simulink library "Trajectory"  (R2016a)
settings: Solver=ode45  StartTime=0.0  StopTime=10.0  RelTol=1e-3
settings Model: Creator=Felipe  LastModifiedBy=md13acp
settings DataIOCC: LimitDataPoints=on  SaveFormat=Array
settings DebuggingCC: UnderspecifiedInitializationDetection=Classic  MergeDetectMultiDrivingBlocksExec=none  SolverPrmCheckMsg=warning  StateNameClashWarn=warning
settings HardwareCC: ProdBitPerPointer=32  ProdLargestAtomicFloat=None  ProdIntDivRoundTo=Undefined  ProdEndianess=Unspecified  ProdWordSize=32  ProdHWDeviceType=32-bit Generic
settings ModelReferenceCC: PropagateSignalLabelsOutOfModel=off
settings ConfigComp: CovModelRefEnable=Off

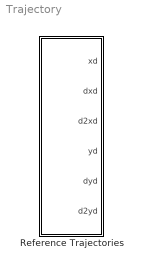
== system Trajectory ==
  Reference Trajectories : Subsystem  mask(Reference Trajectories){trajectory_type=2, wf=0.10, raio_ref_1=1, delta_raio=-0.1, t_delta_raio=60, xd=[2, 3]}
      mask prompts: trajectory_type "Trajectory type: 1=Circle, 2=Eight, 3=Line, 4=Fixed Point"; wf "Angular speed for circle and eight [rad/s]"; raio_ref_1 "Radius for circle and eight (each side) [m]"; delta_raio "Radius variation (circle only)"; t_delta_raio "Time between radius variation (circle only) [s]"; xd "Goal position (for fixed point only) (1x2)"
      mask help: Generates reference values of position, velocity and acceleration.
      mask Help:
      | Generates reference values of position, velocity and acceleration.
      | This block is intended to be used with mobile robot trajectory tracking kinematic controller.
      | 
      | Available references:
      | - Circular trajectory with 2 different radius;
      | - Eight-shape trajectory;
      | - Linear trajectory;
      | - Fixed point.
      | 
      | 
      | <b> Parameters:</b>
      | 
      | Trajectory type: 1=Circle, 2=Eight, 3=Line, 4=Fixed Point
      | Angular speed for circle and eight (1x1) [rad/s]
      | Radius for circle and eight (each side) (1x1)[m]
      | Radius variation (circle only) delta_raio (1x1) [m]
      | Time between radius variation (circle only) (1x1) [s]
      | 
      | <b> Outputs: </b>
      | 
      | xd: desired robot position [m] in x axis;
      | dxd: desired robot speed [m/s] in x axis;
      | d2xd: desired robot acceleration [m/s^2] in x axis;
      | yd: desired robot position [m] in y axis;
      | dyd: desired robot speed [m/s] in y axis;
      | d2yd: desired robot acceleration [m/s^2] in y axis;

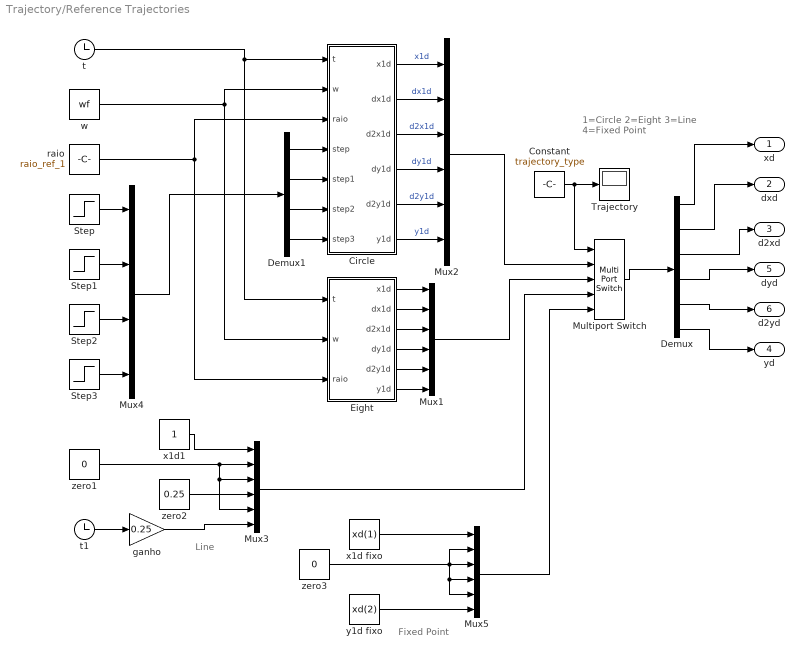
== system Trajectory/Reference Trajectories ==
  note: Fixed Point
  note: Line
  note: 1=Circle
      | 2=Eight
      | 3=Line
      | 4=Fixed Point
  Circle : Subsystem
  Constant : Constant  Value=trajectory_type
  Demux : Demux  Outputs=6
  Demux1 : Demux
  Eight : Subsystem
  Multiport Switch : MultiPortSwitch  Inputs=4  SaturateOnIntegerOverflow=on
  Mux{1..3,5} (4 alike) : Mux  Inputs=6
  Mux4 : Mux
  Step : Step  Time=t_delta_raio  After=delta_raio  SampleTime=0
  Step1 : Step  Time=t_delta_raio*2  After=-delta_raio  SampleTime=0
  Step2 : Step  Time=t_delta_raio*3  After=delta_raio  SampleTime=0
  Step3 : Step  Time=t_delta_raio*4  After=-delta_raio  SampleTime=0
  Trajectory : Display
      settings: Format=decimal (Stored Integer)
  ganho : Gain  Gain=0.25  SaturateOnIntegerOverflow=on  OutDataTypeStr=Inherit: Same as input  ParamDataTypeStr=Inherit: Same as input
  raio : Constant  Value=raio_ref_1
  t : Clock
  t1 : Clock
  w : Constant  Value=wf
  x1d fixo : Constant  Value=xd(1)
  x1d1 : Constant
  y1d fixo : Constant  Value=xd(2)
  zero1 : Constant  Value=0
  zero2 : Constant  Value=0.25
  zero3 : Constant  Value=0
  xd : Outport
  dxd : Outport  Port=2
  d2xd : Outport  Port=3
  yd : Outport  Port=4
  dyd : Outport  Port=5
  d2yd : Outport  Port=6
  wires:
  zero3/1 -> Mux5/5, Mux5/4, Mux5/2, Mux5/3
  x1d fixo/1 -> Mux5/1
  y1d fixo/1 -> Mux5/6
  Mux5/1 -> Multiport Switch/5
  Mux3/1 -> Multiport Switch/4
  Multiport Switch/1 -> Demux/1
  Mux4/1 -> Demux1/1
  Demux1/4 -> Circle/7(step3)
  Demux1/3 -> Circle/6(step2)
  Demux1/2 -> Circle/5(step1)
  Demux1/1 -> Circle/4(step)
  Step3/1 -> Mux4/4
  Step2/1 -> Mux4/3
  Step1/1 -> Mux4/2
  Step/1 -> Mux4/1
  zero2/1 -> Mux3/4
  ganho/1 -> Mux3/6
  zero1/1 -> Mux3/5, Mux3/3, Mux3/2
  t1/1 -> ganho/1
  x1d1/1 -> Mux3/1
  Eight/6(y1d) -> Mux1/6
  Eight/5(d2y1d) -> Mux1/5
  Eight/4(dy1d) -> Mux1/4
  Eight/3(d2x1d) -> Mux1/3
  Eight/2(dx1d) -> Mux1/2
  Eight/1(x1d) -> Mux1/1
  Circle/6(y1d) -> Mux2/6  "y1d"
  Circle/5(d2y1d) -> Mux2/5  "d2y1d"
  Circle/4(dy1d) -> Mux2/4  "dy1d"
  Circle/3(d2x1d) -> Mux2/3  "d2x1d"
  Circle/2(dx1d) -> Mux2/2  "dx1d"
  Circle/1(x1d) -> Mux2/1  "x1d"
  Demux/6 -> yd/1
  Demux/5 -> d2yd/1
  Demux/4 -> dyd/1
  Demux/3 -> d2xd/1
  Demux/2 -> dxd/1
  Demux/1 -> xd/1
  Constant/1 -> Trajectory/1, Multiport Switch/1
  Mux2/1 -> Multiport Switch/2
  Mux1/1 -> Multiport Switch/3
  w/1 -> Eight/2(w), Circle/2(w)
  raio/1 -> Eight/3(raio), Circle/3(raio)
  t/1 -> Eight/1(t), Circle/1(t)

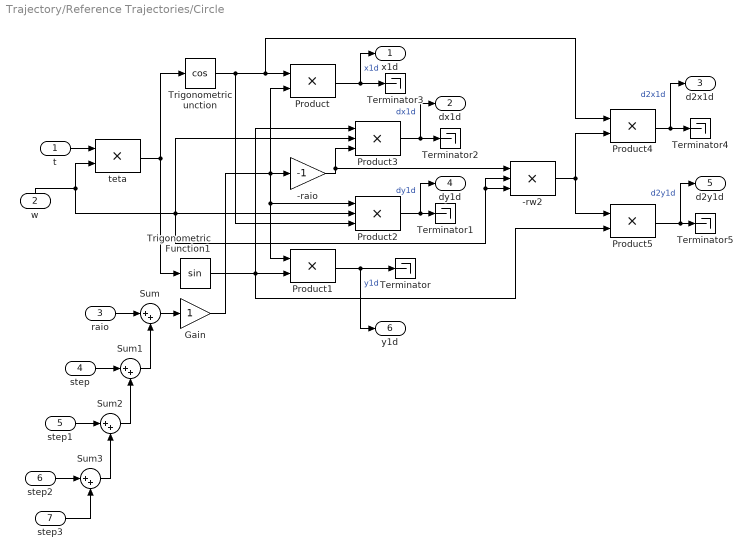
== system Trajectory/Reference Trajectories/Circle ==
  t : Inport
  w : Inport  Port=2
  raio : Inport  Port=3
  step : Inport  Port=4
  step1 : Inport  Port=5
  step2 : Inport  Port=6
  step3 : Inport  Port=7
  -raio : Gain  Gain=-1  SaturateOnIntegerOverflow=on  OutDataTypeStr=Inherit: Same as input  ParamDataTypeStr=Inherit: Same as input
  -rw2 : Product  Inputs=3  SaturateOnIntegerOverflow=on  OutDataTypeStr=Inherit: Same as first input
  Gain : Gain  SaturateOnIntegerOverflow=on  OutDataTypeStr=Inherit: Same as input  ParamDataTypeStr=Inherit: Same as input
  Product{,1,4..5} (4 alike) : Product  SaturateOnIntegerOverflow=on  OutDataTypeStr=Inherit: Same as first input
  Product2 : Product  Inputs=3  SaturateOnIntegerOverflow=on  OutDataTypeStr=Inherit: Same as first input
  Product3 : Product  Inputs=3  SaturateOnIntegerOverflow=on  OutDataTypeStr=Inherit: Same as first input
  Sum{,1..3} (4 alike) : Sum  Inputs=|++  SaturateOnIntegerOverflow=on
  Terminator{,1..5} (6 alike) : Terminator
  Trigonometric Function1 : Trigonometry
  Trigonometric unction : Trigonometry  Operator=cos
  teta : Product  SaturateOnIntegerOverflow=on  OutDataTypeStr=Inherit: Same as first input
  x1d : Outport
  dx1d : Outport  Port=2
  d2x1d : Outport  Port=3
  dy1d : Outport  Port=4
  d2y1d : Outport  Port=5
  y1d : Outport  Port=6
  wires:
  step3/1 -> Sum3/2
  step2/1 -> Sum3/1
  step1/1 -> Sum2/1
  step/1 -> Sum1/1
  raio/1 -> Sum/1
  t/1 -> teta/1
  Sum3/1 -> Sum2/2
  Sum2/1 -> Sum1/2
  Sum1/1 -> Sum/2
  Sum/1 -> Gain/1
  Gain/1 -> Product/2, Product2/1, Product1/1, -raio/1
  Product5/1 -> d2y1d/1, Terminator5/1  "d2y1d"
  Product4/1 -> d2x1d/1, Terminator4/1  "d2x1d"
  -rw2/1 -> Product5/1, Product4/2
  -raio/1 -> -rw2/1, Product3/3
  Product3/1 -> dx1d/1, Terminator2/1  "dx1d"
  Product2/1 -> dy1d/1, Terminator1/1  "dy1d"
  teta/1 -> Trigonometric Function1/1, Trigonometric unction/1
  Product1/1 -> Terminator/1, y1d/1  "y1d"
  Product/1 -> Terminator3/1, x1d/1  "x1d"
  w/1 -> teta/2, Product3/2, -rw2/3, -rw2/2, Product2/2
  Trigonometric Function1/1 -> Product5/2, Product3/1, Product1/2
  Trigonometric unction/1 -> Product/1, Product4/1, Product2/3

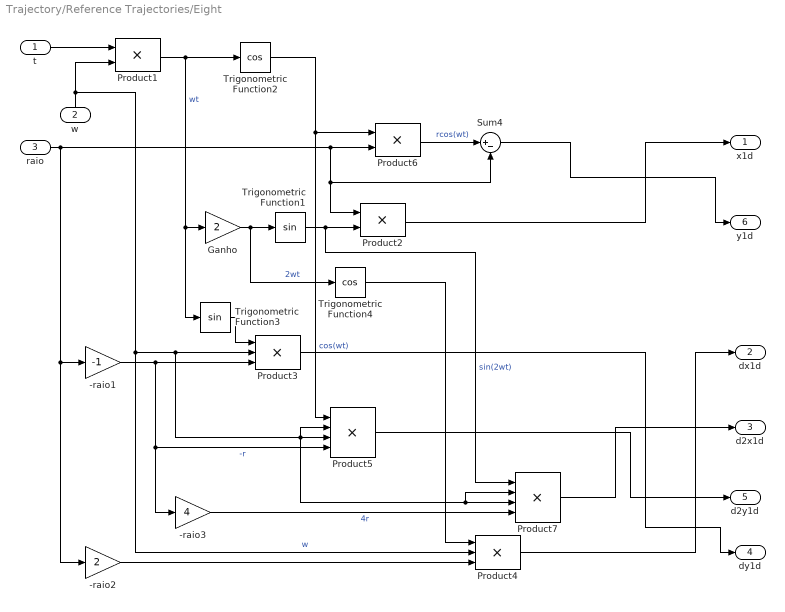
== system Trajectory/Reference Trajectories/Eight ==
  t : Inport
  w : Inport  Port=2
  raio : Inport  Port=3
  -raio1 : Gain  Gain=-1  SaturateOnIntegerOverflow=on  OutDataTypeStr=Inherit: Same as input  ParamDataTypeStr=Inherit: Same as input
  -raio2 : Gain  Gain=2  SaturateOnIntegerOverflow=on  OutDataTypeStr=Inherit: Same as input  ParamDataTypeStr=Inherit: Same as input
  -raio3 : Gain  Gain=4  SaturateOnIntegerOverflow=on  OutDataTypeStr=Inherit: Same as input  ParamDataTypeStr=Inherit: Same as input
  Ganho : Gain  Gain=2  SaturateOnIntegerOverflow=on  OutDataTypeStr=Inherit: Same as input  ParamDataTypeStr=Inherit: Same as input
  Product1 : Product  SaturateOnIntegerOverflow=on  OutDataTypeStr=Inherit: Same as first input
  Product2 : Product  SaturateOnIntegerOverflow=on  OutDataTypeStr=Inherit: Same as first input
  Product3 : Product  Inputs=3  SaturateOnIntegerOverflow=on  OutDataTypeStr=Inherit: Same as first input
  Product4 : Product  Inputs=3  SaturateOnIntegerOverflow=on  OutDataTypeStr=Inherit: Same as first input
  Product5 : Product  Inputs=4  SaturateOnIntegerOverflow=on  OutDataTypeStr=Inherit: Same as first input
  Product6 : Product  SaturateOnIntegerOverflow=on  OutDataTypeStr=Inherit: Same as first input
  Product7 : Product  Inputs=4  SaturateOnIntegerOverflow=on  OutDataTypeStr=Inherit: Same as first input
  Sum4 : Sum  Inputs=|+-  SaturateOnIntegerOverflow=on
  Trigonometric Function1 : Trigonometry
  Trigonometric Function2 : Trigonometry  Operator=cos
  Trigonometric Function3 : Trigonometry
  Trigonometric Function4 : Trigonometry  Operator=cos
  x1d : Outport
  dx1d : Outport  Port=2
  d2x1d : Outport  Port=3
  dy1d : Outport  Port=4
  d2y1d : Outport  Port=5
  y1d : Outport  Port=6
  wires:
  Product5/1 -> d2y1d/1
  Product7/1 -> d2x1d/1
  Product3/1 -> dy1d/1
  Product4/1 -> dx1d/1
  Sum4/1 -> y1d/1
  Product2/1 -> x1d/1
  -raio3/1 -> Product7/4  "4r"
  Trigonometric Function4/1 -> Product4/1
  -raio2/1 -> Product4/3
  -raio1/1 -> -raio3/1, Product5/4, Product3/3  "-r"
  Trigonometric Function3/1 -> Product3/1
  Trigonometric Function1/1 -> Product7/1, Product2/2  "sin(2wt)"
  Ganho/1 -> Trigonometric Function4/1, Trigonometric Function1/1  "2wt"
  Product6/1 -> Sum4/1  "rcos(wt)"
  Trigonometric Function2/1 -> Product5/1, Product6/1  "cos(wt)"
  raio/1 -> -raio2/1, -raio1/1, Product2/1, Sum4/2, Product6/2
  Product1/1 -> Trigonometric Function3/1, Ganho/1, Trigonometric Function2/1  "wt"
  w/1 -> Product7/2, Product7/3, Product5/2, Product5/3, Product3/2, Product4/2, Product1/2  "w"
  t/1 -> Product1/1
